simulink model "IBS_phase7"  (R2026a)
settings: Solver=ode45  StopTime=6000  MaxStep=5  AbsTol=1e-3
undefined symbols (not defined in the file or in its folder): juliandate
libraries: simulink x1, aerolibcubesatveh x1
settings Model: Creator=LENOVO  LastModifiedBy=LENOVO

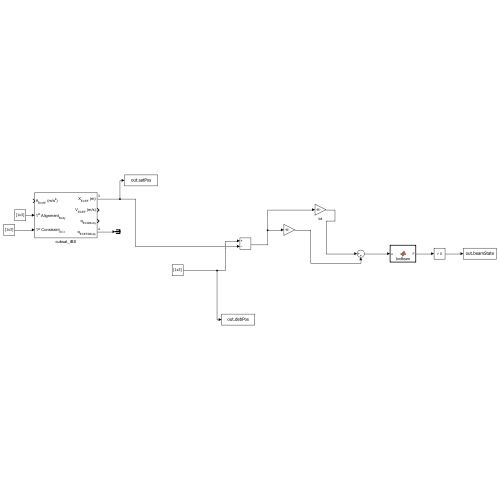
[thumbnail: Simulink's stored preview of the top-level diagram]
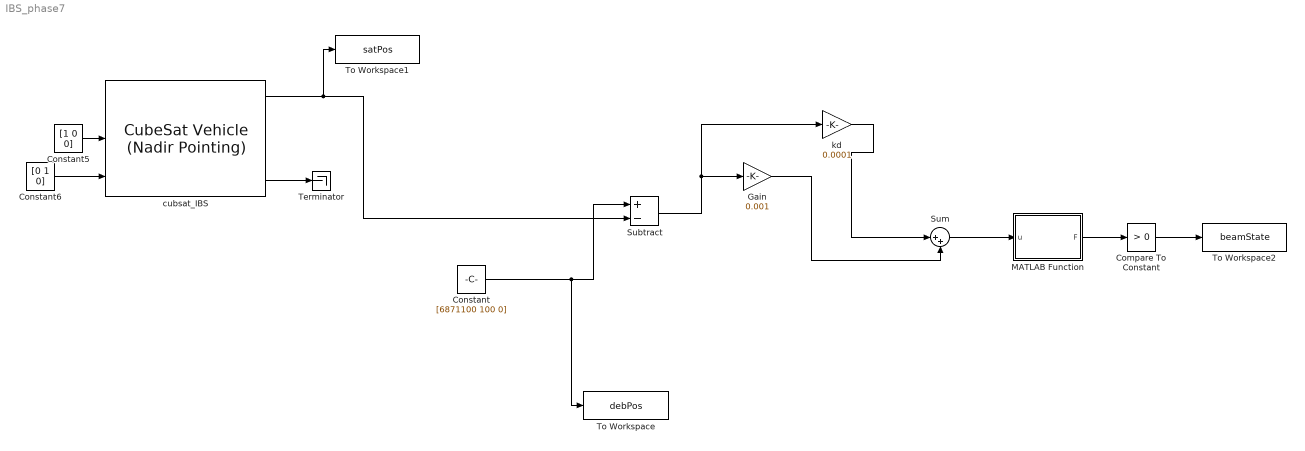
== system IBS_phase7 ==
  Compare To Constant : simulink/Logic and Bit Operations/Compare To Constant  relop=>  const=0  OutDataTypeStr=boolean
  Constant : Constant  Value=[6871100 100 0]  VectorParams1D=off
  Constant5 : Constant  Value=[1 0 0]
  Constant6 : Constant  Value=[0 1 0]
  Gain : Gain  Gain=0.001
  MATLAB Function : MATLAB Function  TreatAsAtomicUnit=on
  Subtract : Sum  Inputs=+-
  Sum : Sum  Inputs=|++
  Terminator : Terminator
  To Workspace : ToWorkspace  VariableName=debPos  SampleTime=-1
      settings: Save2DSignal=2-D array (concatenate along first dimension)
  To Workspace1 : ToWorkspace  VariableName=satPos  SampleTime=-1
      settings: Save2DSignal=2-D array (concatenate along first dimension)
  To Workspace2 : ToWorkspace  VariableName=beamState  SampleTime=-1
      settings: Save2DSignal=2-D array (concatenate along first dimension)
  cubsat_IBS : aerolibcubesatveh/CubeSat Vehicle (Nadir Pointing)  sim_t0=juliandate(2019, 1, 4, 12, 0, 0)  method=Keplerian Orbital Elements  epoch=juliandate(2000, 1, 1, 12, 0, 0)  a=6878137  ecc=0  incl=0  omega=0  argp=0  nu=0  truelon=0  arglat=0  lonper=0  r_eci=[0 0 0]  v_eci=[0 0 0]  r_ecef=[0 0 0]  v_ecef=[0 0 0]  lla=[0 0 0]  v_ned=[0 0 0]  euler=[0 0 0]  pqr=[0 0 -0.05168]  pointingMode=Custom Pointing  firstAlignExt=Input port  firstAlign=[0 0 1]  secondAlignExt=Dialog  secondAlign=[0 1 0]  constraintCoord=ECI Axes  firstRefExt=Input port  firstRef=[1 0 0]  secondRefExt=Dialog  secondRef=[0 0 1]  missionRTSource=Dialog  missionRT=6*60*60  missionGS=[42, -71]  missionTOICheck=on  missionTOI=[]  missionEta=55
      settings: LibrarySourceBlock=|
      | aerolibcubesatveh/CubeSat Vehicle
      | (Custom Pointing)
  kd : Gain  Gain=0.0001
  wires:
  Sum/1 -> MATLAB Function/1(u)
  Subtract/1 -> Gain/1, kd/1
  Gain/1 -> Sum/2
  kd/1 -> Sum/1
  MATLAB Function/1(F) -> Compare To Constant/1
  Compare To Constant/1 -> To Workspace2/1
  Constant5/1 -> cubsat_IBS/2
  cubsat_IBS/1 -> To Workspace1/1, Subtract/2
  Constant6/1 -> cubsat_IBS/3
  Constant/1 -> Subtract/1, To Workspace/1
  cubsat_IBS/4 -> Terminator/1

== matlab function IBS_phase7/MATLAB Function ==
  data: u input; F output
function F = IonBeam(u)

F = 0.02*norm(u);
end
